simulink model "Modul_PV_V2"  (R2023a)
settings: Solver=ode3  StartTime=0.0  StopTime=3  RelTol=1e-3
libraries: simulink x3, SignalEditorBlockLib x2
settings Model: Creator=lucea  LastModifiedBy=lucea
settings DebuggingCC: AlgebraicLoopMsg=none

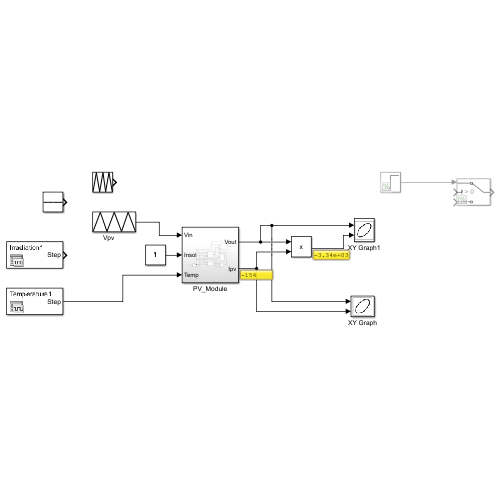
[thumbnail: Simulink's stored preview of the top-level diagram]
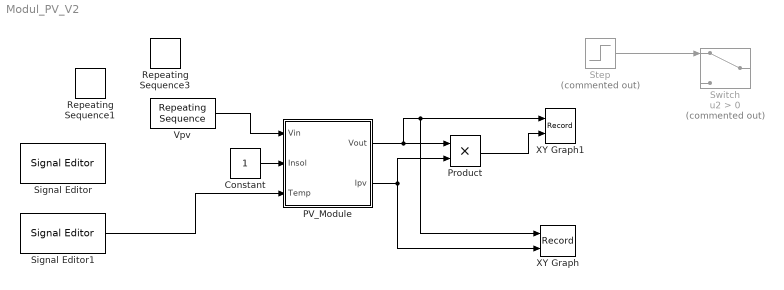
== system Modul_PV_V2 ==
  Constant : Constant
  PV_Module : Subsystem
  Product : Product
  Repeating Sequence1 : simulink/Sources/Repeating Sequence  rep_seq_t=[0 1 2 3 4 5]  rep_seq_y=[22.4 22.4 22.4 22.4 22.4 22.4]
  Repeating Sequence3 : simulink/Sources/Repeating Sequence  rep_seq_t=[0 1 2]  rep_seq_y=[0.1 21.4 0.1]
  Signal Editor : SignalEditorBlockLib/Signal Editor  FileName=irradinput.mat  ActiveScenario=Irradiation1  ActiveSignal=Step  IsBus=off  OutputBusObjectStr=Bus: BusObject  SampleTime=0  Interpolate=off  ZeroCross=off  OutputAfterFinalValue=Setting to zero  Unit=inherit  PreserveSignalName=on  ApplySigPropsToAllScenarios=on
  Signal Editor1 : SignalEditorBlockLib/Signal Editor  FileName=temp.mat  ActiveScenario=Temperature1  ActiveSignal=Step  IsBus=off  OutputBusObjectStr=Bus: BusObject  SampleTime=0  Interpolate=off  ZeroCross=off  OutputAfterFinalValue=Setting to zero  Unit=inherit  PreserveSignalName=on  ApplySigPropsToAllScenarios=on
  Step : Step  Commented=on  After=200  SampleTime=0
  Switch : Switch  Commented=on  Criteria=u2 > Threshold  SaturateOnIntegerOverflow=off  InputSameDT=off
  "Vpv      " : simulink/Sources/Repeating Sequence  rep_seq_t=[0 1 2]  rep_seq_y="[0.1  21.6 0.1]"
  XY Graph : Record  FileSettingsInternal="{\"entries\":[{\"content\":{\"excelSettings\":{\"content\":{},\"type\":\"Streamout.ExcelSettings\"}},\"type\":\"Streamout.FileSettingStorage\",\"uuid\":\"\"}],\"packageUris\":[\"http:\\/\\/schema.mathworks.com\\/mf0\\/streamout_blocks\\/R2020a\"],\"version\":\"1.0\"}"  Layout=[1 1]  SignalsInternal="{\"entries\":[{\"content\":{\"signals\":[{\"content\":{\"blockPath\":[],\"dimensions\":[1],\"domain\":\"\",\"lineColor\":\"#a2142f\",\"plots\":[1],\"port\":1,\"sid\":[\"\"],\"signalID\":1045,\"signalName\":\"PV_Module:1\"},\"type\":\"RecordBlkView.Signal\",\"uuid\":\"\"},{\"content\":{\"blockPath\":[],\"dimensions\":[1],\"domain\":\"\",\"lineColor\":\"#139fff\",\"plots\":[1],\"port\":2,\"sid\":[\"\"],\"signalID\":1049,\"signalName\":\"PV_Module:2\"},\"type\":\"RecordBlkView.Signal\",\"uuid\":\"\"}]},\"type\":\"RecordBlkView.InputSignals\",\"uuid\":\"\"}],\"packageUris\":[\"http:\\/\\/schema.mathworks.com\\/mf0\\/streamout_blocks\\/R2020a\"],\"version\":\"1.0\"}"  VisualizationBindings="{\"xyplotplugin\":{\"info\":[{\"series\":[{\"bindingParametersList\":[{\"parameter\":\"X-Axis\",\"signalID\":1045,\"signalName\":\"PV_Module:1\"},{\"parameter\":\"Y-Axis\",\"signalID\":1049,\"signalName\":\"PV_Module:2\"}],\"seriesID\":20498}],\"subplotID\":1}]}}"  CompatibilityTag=XY
  XY Graph1 : Record  FileSettingsInternal="{\"entries\":[{\"content\":{\"excelSettings\":{\"content\":{},\"type\":\"Streamout.ExcelSettings\"}},\"type\":\"Streamout.FileSettingStorage\",\"uuid\":\"\"}],\"packageUris\":[\"http:\\/\\/schema.mathworks.com\\/mf0\\/streamout_blocks\\/R2020a\"],\"version\":\"1.0\"}"  Layout=[1 1]  SignalsInternal="{\"entries\":[{\"content\":{\"signals\":[{\"content\":{\"blockPath\":[],\"dimensions\":[1],\"domain\":\"\",\"lineColor\":\"#a2142f\",\"plots\":[1],\"port\":1,\"sid\":[\"\"],\"signalID\":1053,\"signalName\":\"PV_Module:1\"},\"type\":\"RecordBlkView.Signal\",\"uuid\":\"\"},{\"content\":{\"blockPath\":[],\"dimensions\":[1],\"domain\":\"\",\"lineColor\":\"#139fff\",\"plots\":[1],\"port\":2,\"sid\":[\"\"],\"signalID\":1057,\"signalName\":\"Product\"},\"type\":\"RecordBlkView.Signal\",\"uuid\":\"\"}]},\"type\":\"RecordBlkView.InputSignals\",\"uuid\":\"\"}],\"packageUris\":[\"http:\\/\\/schema.mathworks.com\\/mf0\\/streamout_blocks\\/R2020a\"],\"version\":\"1.0\"}"  VisualizationBindings="{\"xyplotplugin\":{\"info\":[{\"series\":[{\"bindingParametersList\":[{\"parameter\":\"X-Axis\",\"signalID\":1053,\"signalName\":\"PV_Module:1\"},{\"parameter\":\"Y-Axis\",\"signalID\":1057,\"signalName\":\"Product\"}],\"seriesID\":1089}],\"subplotID\":1}]}}"  CompatibilityTag=XY  st=-1
  wires:
  Step/1 -> Switch/1
  Signal Editor1/1 -> PV_Module/3(Temp)
  PV_Module/2(Ipv) -> XY Graph/2, Product/2
  PV_Module/1(Vout) -> XY Graph/1, XY Graph1/1, Product/1
  Product/1 -> XY Graph1/2
  "Vpv      "/1 -> PV_Module/1(Vin)
  Constant/1 -> PV_Module/2(Insol)

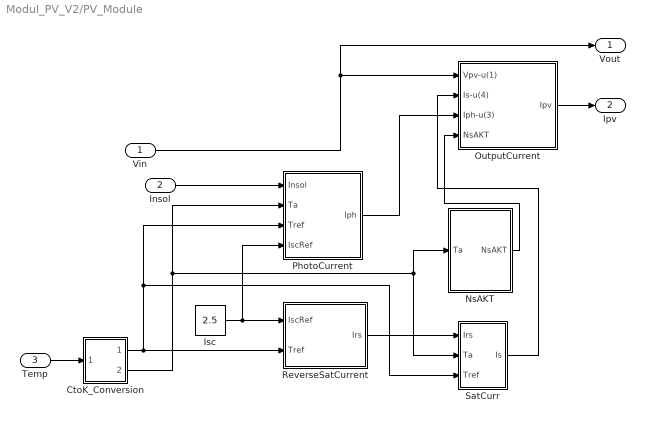
== system Modul_PV_V2/PV_Module ==
  Vin : Inport
  Insol : Inport  Port=2
  Temp : Inport  Port=3
  CtoK_Conversion : Subsystem
  Isc : Constant  Value=2.5
  NsAKT : Subsystem
  OutputCurrent : Subsystem
  PhotoCurrent : Subsystem
  ReverseSatCurrent : Subsystem
  SatCurr : Subsystem
  Vout : Outport
  Ipv : Outport  Port=2
  wires:
  CtoK_Conversion/1(Tref_K) -> PhotoCurrent/3(Tref), SatCurr/3(Tref), ReverseSatCurrent/2(Tref)
  PhotoCurrent/1(Iph) -> OutputCurrent/3(Iph-u(3))
  Insol/1 -> PhotoCurrent/1(Insol)
  NsAKT/1(NsAKT) -> OutputCurrent/4(NsAKT)
  SatCurr/1(Is) -> OutputCurrent/2(Is-u(4))
  CtoK_Conversion/2(Ta_K) -> PhotoCurrent/2(Ta), SatCurr/2(Ta), NsAKT/1(Ta)
  Vin/1 -> Vout/1, OutputCurrent/1(Vpv-u(1))
  Temp/1 -> CtoK_Conversion/1(Top)
  ReverseSatCurrent/1(Irs) -> SatCurr/1(Irs)
  OutputCurrent/1(Ipv) -> Ipv/1
  Isc/1 -> PhotoCurrent/4(IscRef), ReverseSatCurrent/1(IscRef)

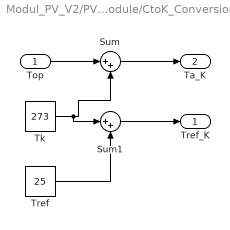
== system Modul_PV_V2/PV_Module/CtoK_Conversion ==
  Top : Inport
  Sum : Sum  Inputs=|++
  Sum1 : Sum  Inputs=|++
  Tk : Constant  Value=273
  Tref : Constant  Value=25
  Tref_K : Outport
  Ta_K : Outport  Port=2
  wires:
  Tk/1 -> Sum/2, Sum1/1
  Tref/1 -> Sum1/2
  Sum/1 -> Ta_K/1
  Sum1/1 -> Tref_K/1
  Top/1 -> Sum/1

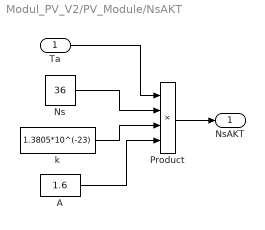
== system Modul_PV_V2/PV_Module/NsAKT ==
  Ta : Inport
  A : Constant  Value=1.6
  Ns : Constant  Value=36
  Product : Product  Inputs=4
  k : Constant  Value=1.3805*10^(-23)
  NsAKT : Outport
  wires:
  Ta/1 -> Product/1
  Ns/1 -> Product/2
  Product/1 -> NsAKT/1
  A/1 -> Product/4
  k/1 -> Product/3

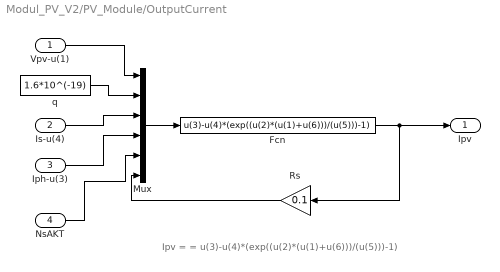
== system Modul_PV_V2/PV_Module/OutputCurrent ==
  note: Ipv = = u(3)-u(4)*(exp((u(2)*(u(1)+u(6)))/(u(5)))-1)
  Vpv-u(1) : Inport
  Is-u(4) : Inport  Port=2
  Iph-u(3) : Inport  Port=3
  NsAKT : Inport  Port=4
  Fcn : Fcn  Expr=u(3)-u(4)*(exp((u(2)*(u(1)+u(6)))/(u(5)))-1)
  Mux : Mux  Inputs=6
  Rs : Gain  Gain=0.1
  q : Constant  Value=1.6*10^(-19)
  Ipv : Outport
  wires:
  Vpv-u(1)/1 -> Mux/1
  Is-u(4)/1 -> Mux/3
  Fcn/1 -> Ipv/1, Rs/1
  q/1 -> Mux/2
  Rs/1 -> Mux/6
  Mux/1 -> Fcn/1
  Iph-u(3)/1 -> Mux/4
  NsAKT/1 -> Mux/5

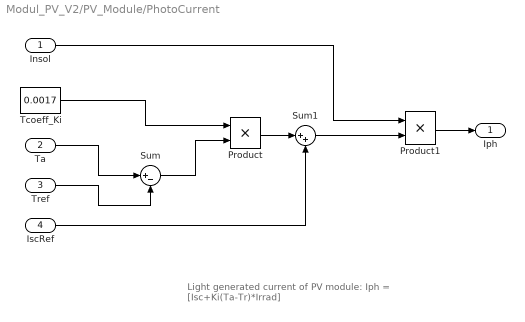
== system Modul_PV_V2/PV_Module/PhotoCurrent ==
  note: Light generated current of PV module:
      | Iph = [Isc+Ki(Ta-Tr)*Irrad]
  Insol : Inport
  Ta : Inport  Port=2
  Tref : Inport  Port=3
  IscRef : Inport  Port=4
  Product : Product
  Product1 : Product
  Sum : Sum  Inputs=|+-
  Sum1 : Sum  Inputs=|++
  Tcoeff_Ki : Constant  Value=0.0017
  Iph : Outport
  wires:
  IscRef/1 -> Sum1/2
  Insol/1 -> Product1/1
  Tcoeff_Ki/1 -> Product/1
  Ta/1 -> Sum/1
  Sum/1 -> Product/2
  Product/1 -> Sum1/1
  Sum1/1 -> Product1/2
  Product1/1 -> Iph/1
  Tref/1 -> Sum/2

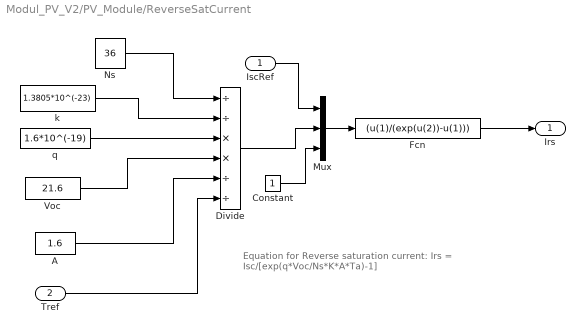
== system Modul_PV_V2/PV_Module/ReverseSatCurrent ==
  note: Equation for Reverse saturation current:
      | Irs = Isc/[exp(q*Voc/Ns*K*A*Ta)-1]
  IscRef : Inport
  Tref : Inport  Port=2
  A : Constant  Value=1.6
  Constant : Constant
  Divide : Product  Inputs=//**//
  Fcn : Fcn  Expr=(u(1)/(exp(u(2))-u(1)))
  Mux : Mux  Inputs=3
  Ns : Constant  Value=36
  Voc : Constant  Value=21.6
  k : Constant  Value=1.3805*10^(-23)
  q : Constant  Value=1.6*10^(-19)
  Irs : Outport
  wires:
  Ns/1 -> Divide/1
  Voc/1 -> Divide/4
  k/1 -> Divide/2
  Constant/1 -> Mux/3
  Divide/1 -> Mux/2
  Fcn/1 -> Irs/1
  Mux/1 -> Fcn/1
  A/1 -> Divide/5
  IscRef/1 -> Mux/1
  Tref/1 -> Divide/6
  q/1 -> Divide/3

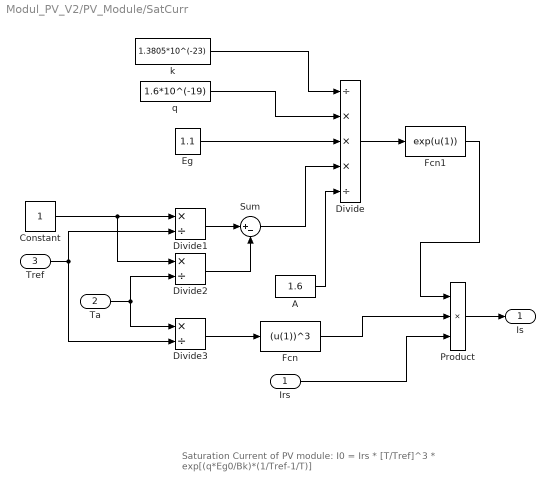
== system Modul_PV_V2/PV_Module/SatCurr ==
  note: Saturation Current of PV module:
      | I0 = Irs * [T/Tref]^3 * exp[(q*Eg0/Bk)*(1/Tref-1/T)]
  Irs : Inport
  Ta : Inport  Port=2
  Tref : Inport  Port=3
  A : Constant  Value=1.6
  Constant : Constant
  Divide : Product  Inputs=/***/
  Divide1 : Product  Inputs=*/
  Divide2 : Product  Inputs=*/
  Divide3 : Product  Inputs=*/
  Eg : Constant  Value=1.1
  Fcn : Fcn  Expr=(u(1))^3
  Fcn1 : Fcn  Expr=exp(u(1))
  Product : Product  Inputs=3
  Sum : Sum  Inputs=|+-
  k : Constant  Value=1.3805*10^(-23)
  q : Constant  Value=1.6*10^(-19)
  Is : Outport
  wires:
  Fcn/1 -> Product/2
  Fcn1/1 -> Product/1
  Ta/1 -> Divide3/1, Divide2/2
  Tref/1 -> Divide1/2, Divide3/2
  Divide1/1 -> Sum/1
  Constant/1 -> Divide2/1, Divide1/1
  Divide/1 -> Fcn1/1
  A/1 -> Divide/5
  Eg/1 -> Divide/3
  Sum/1 -> Divide/4
  k/1 -> Divide/1
  Irs/1 -> Product/3
  Product/1 -> Is/1
  Divide2/1 -> Sum/2
  q/1 -> Divide/2
  Divide3/1 -> Fcn/1
